simulink model "PMSM_FOC_Average_Inveter"  (R2020b)
settings: Solver=FixedStepAuto  StartTime=0.0  StopTime=10  FixedStep=Fixed_Step_Size  RelTol=1e-3
model workspace (MAT data in the model file):
  wc : Simulink.Parameter (value not decoded)
values from neighbouring files (symbols this model uses):
  Angle = 1.0    [Motor_Control_Data.sldd]
  Cosine_table = 1.0 0.99999529 0.99999058 0.99998587 0.99998116 0.99996704 0.99995291 0.99993885 0.99992472 0.99990118 0.99987763 0.99985409 0.9998306 0.99979764 0.99976468 0.99973178 0.99969882 0.99965644 0.99961412 0.99957174 0.99952942 0.99947762 0.99942589 0.99937415 0.99932235 0.9992612 0.99920005 0.99913889 0.99907768 0.99900717 0.99893659 0.99886602 0.99879545 0.99871546 0.99863547 0.99855554 0.99847555 0.    [Motor_Control_Data.sldd]
  Fixed_Step_Size = 1.0E-5    [Motor_Control_Data.sldd]
  Flux = 0.1125    [Motor_Control_Data.sldd]
  ID_Ki = 48.0    [Motor_Control_Data.sldd]
  ID_Kp = 0.84    [Motor_Control_Data.sldd]
  IQ_Ki = 48.0    [Motor_Control_Data.sldd]
  IQ_Kp = 1.869    [Motor_Control_Data.sldd]
  Ld = 0.00014    [Motor_Control_Data.sldd]
  Lq = 0.0003115    [Motor_Control_Data.sldd]
  MTPA_Te_Min = 0.0    [Motor_Control_Data.sldd]
  Pole_Pairs = 4.0    [Motor_Control_Data.sldd]
  PWM_Frequency = 10000.0    [Motor_Control_Data.sldd]
  Sine_table = 0.0 0.0015339879 0.0030679768 0.0046019657 0.0061359555 0.0076698866 0.0092038177 0.010737749 0.012271681 0.013805497 0.015339312 0.016873131 0.018406944 0.019940587 0.021474229 0.023007872 0.024541514 0.026074925 0.027608337 0.029141748 0.03067516 0.032208283 0.033741407 0.035274528 0.036807653 0.038340431 0.039873205 0.04140598 0.042938754 0.04447113 0.046003502 0.047535874 0.049068246 0.0506001    [Motor_Control_Data.sldd]
  Speed_Ki = 10.809    [Motor_Control_Data.sldd]
  Speed_Kp = 0.08    [Motor_Control_Data.sldd]
  Speed_PI_OutputMax = 700.0    [Motor_Control_Data.sldd]
  Speed_PI_OutputMin = -700.0    [Motor_Control_Data.sldd]
  TorqueMode = 0.0    [Motor_Control_Data.sldd]
undefined symbols (not defined in the file or in its folder): Angle_offset, DiscIntNeverNeededParam, FluxWeak_Enable, FluxWeak_Idref_max, FluxWeak_Idref_min, FluxWeak_Ki, FluxWeak_Kp, inverter, MTPA_id_table, MTPA_iq_table, MTPA_Te_Max, Over_modulation, sigbuilder_block, SVPWM
libraries: simulink x7, pid_lib x1, mcbplantlib x1, autolibpmsminterior x1
(part 2 of 2)

== system PMSM_FOC_Average_Inveter/Motor_Control/Motor_Control_Function/FOC_Control_100us/FOC/Inverse_Park_Transform ==
  D : Inport
  Q : Inport  Port=2
  Sin_Coefficient : Inport  Port=3
  Cos_Coefficient : Inport  Port=4
  Add1 : Sum  Inputs=+-  OutDataTypeStr=Inherit: Same as first input
  Add2 : Sum  OutDataTypeStr=Inherit: Same as first input
  Cos_Coefficient1 : InportShadow  Port=4
  Product{1..4} (4 alike) : Product  RndMeth=Simplest  OutDataTypeStr=Inherit: Same as first input
  Sin_Coefficient1 : InportShadow  Port=3
  Alpha : Outport  VectorParamsAs1DForOutWhenUnconnected=off
  Beta : Outport  Port=2  VectorParamsAs1DForOutWhenUnconnected=off
  wires:
  Add2/1 -> Beta/1
  Add1/1 -> Alpha/1
  Product3/1 -> Add2/1
  Product4/1 -> Add2/2
  Product1/1 -> Add1/1
  Product2/1 -> Add1/2
  Cos_Coefficient1/1 -> Product4/2
  Sin_Coefficient/1 -> Product2/2
  D/1 -> Product3/1, Product1/1
  Q/1 -> Product2/1, Product4/1
  Sin_Coefficient1/1 -> Product3/2
  Cos_Coefficient/1 -> Product1/2

== system PMSM_FOC_Average_Inveter/Motor_Control/Motor_Control_Function/FOC_Control_100us/FOC/Park_Transform ==
  Alpha : Inport
  Beta : Inport  Port=2
  Sin_Coefficient : Inport  Port=3
  Cos_Coefficient : Inport  Port=4
  Add1 : Sum  OutDataTypeStr=Inherit: Same as first input
  Add2 : Sum  Inputs=-+  OutDataTypeStr=Inherit: Same as first input
  Alpha1 : InportShadow
  Beta1 : InportShadow  Port=2
  Cos_Coefficient1 : InportShadow  Port=4
  Produc3t : Product  RndMeth=Simplest  OutDataTypeStr=Inherit: Same as first input
  Product1 : Product  RndMeth=Simplest  OutDataTypeStr=Inherit: Same as first input
  Product2 : Product  RndMeth=Simplest  OutDataTypeStr=Inherit: Same as first input
  Product4 : Product  RndMeth=Simplest  OutDataTypeStr=Inherit: Same as first input
  Sin_Coefficient1 : InportShadow  Port=3
  D : Outport  VectorParamsAs1DForOutWhenUnconnected=off
  Q : Outport  Port=2  VectorParamsAs1DForOutWhenUnconnected=off
  wires:
  Produc3t/1 -> Add2/1
  Product4/1 -> Add2/2
  Product1/1 -> Add1/1
  Product2/1 -> Add1/2
  Alpha1/1 -> Produc3t/1
  Sin_Coefficient1/1 -> Produc3t/2
  Cos_Coefficient1/1 -> Product4/2
  Beta1/1 -> Product4/1
  Alpha/1 -> Product1/1
  Cos_Coefficient/1 -> Product1/2
  Beta/1 -> Product2/1
  Sin_Coefficient/1 -> Product2/2
  Add1/1 -> D/1
  Add2/1 -> Q/1

== system PMSM_FOC_Average_Inveter/Motor_Control/Motor_Control_Function/FOC_Control_100us/FOC/Q_Current_PI ==
  Reset : Inport
  Bus_voltage : Inport  Port=2
  Current_Command : Inport  Port=3
  Current_Measured : Inport  Port=4
  Add2 : Sum  Inputs=|+-
  IQ_Control : Subsystem
  Vq_voltage : Outport  VectorParamsAs1DForOutWhenUnconnected=off
  wires:
  Current_Command/1 -> Add2/1
  Current_Measured/1 -> Add2/2
  Add2/1 -> IQ_Control/3(Err)  "currentControlError"
  IQ_Control/1(PI_Out) -> Vq_voltage/1
  Reset/1 -> IQ_Control/1(Reset)
  Bus_voltage/1 -> IQ_Control/2(Bus_voltage)

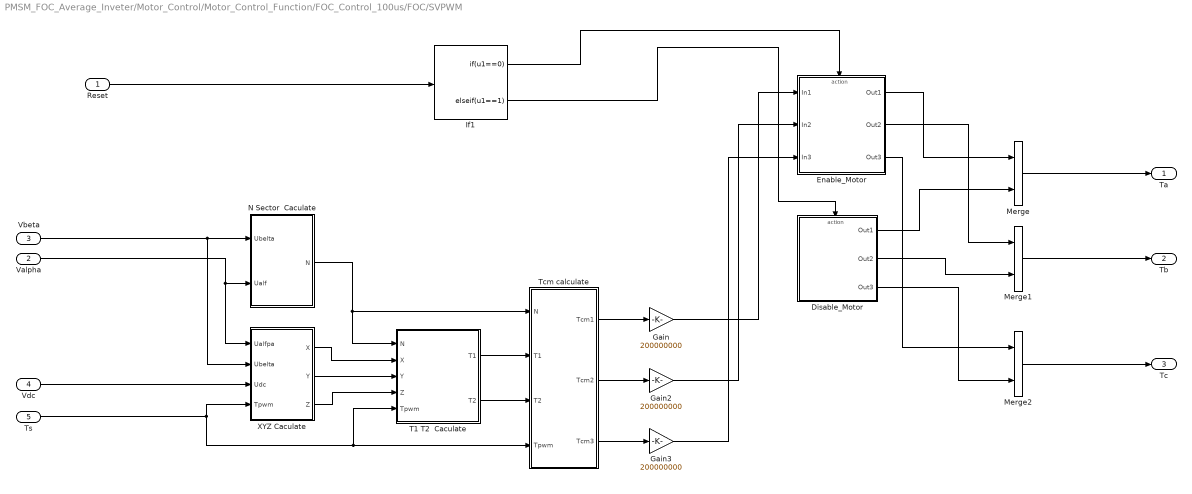
== system PMSM_FOC_Average_Inveter/Motor_Control/Motor_Control_Function/FOC_Control_100us/FOC/SVPWM ==
  Reset : Inport
  Valpha : Inport  Port=2
  Vbeta : Inport  Port=3
  Vdc : Inport  Port=4
  Ts : Inport  Port=5
  Disable_Motor : Subsystem  TreatAsAtomicUnit=on
  Enable_Motor : Subsystem  TreatAsAtomicUnit=on
  Gain : Gain  Gain=200000000
  Gain2 : Gain  Gain=200000000
  Gain3 : Gain  Gain=200000000
  If1 : If  IfExpression=u1==0  ElseIfExpressions=u1==1  ShowElse=off
  Merge : Merge
  Merge1 : Merge
  Merge2 : Merge
  N Sector  Caculate : Subsystem  TreatAsAtomicUnit=on
  T1 T2  Caculate : Subsystem  TreatAsAtomicUnit=on
  Tcm calculate : Subsystem  TreatAsAtomicUnit=on
  XYZ Caculate : Subsystem  TreatAsAtomicUnit=on
  Ta : Outport
  Tb : Outport  Port=2
  Tc : Outport  Port=3
  wires:
  Tcm calculate/2(Tcm2) -> Gain2/1
  Tcm calculate/3(Tcm3) -> Gain3/1
  Tcm calculate/1(Tcm1) -> Gain/1
  T1 T2  Caculate/2(T2) -> Tcm calculate/3(T2)
  XYZ Caculate/1(X) -> T1 T2  Caculate/2(X)
  N Sector  Caculate/1(N) -> T1 T2  Caculate/1(N), Tcm calculate/1(N)
  Vdc/1 -> XYZ Caculate/3(Udc)
  T1 T2  Caculate/1(T1) -> Tcm calculate/2(T1)
  XYZ Caculate/3(Z) -> T1 T2  Caculate/4(Z)
  XYZ Caculate/2(Y) -> T1 T2  Caculate/3(Y)
  Valpha/1 -> N Sector  Caculate/2(Ualf), XYZ Caculate/1(Ualfpa)
  Vbeta/1 -> N Sector  Caculate/1(Ubelta), XYZ Caculate/2(Ubelta)
  Ts/1 -> T1 T2  Caculate/5(Tpwm), Tcm calculate/4(Tpwm), XYZ Caculate/4(Tpwm)
  Gain/1 -> Enable_Motor/1(In1)
  Gain2/1 -> Enable_Motor/2(In2)
  Reset/1 -> If1/1
  If1/1 -> Enable_Motor/Action
  If1/2 -> Disable_Motor/Action
  Gain3/1 -> Enable_Motor/3(In3)
  Enable_Motor/1(Out1) -> Merge/1
  Disable_Motor/1(Out1) -> Merge/2
  Enable_Motor/2(Out2) -> Merge1/1
  Disable_Motor/2(Out2) -> Merge1/2
  Enable_Motor/3(Out3) -> Merge2/1
  Disable_Motor/3(Out3) -> Merge2/2
  Merge/1 -> Ta/1
  Merge1/1 -> Tb/1
  Merge2/1 -> Tc/1

== system PMSM_FOC_Average_Inveter/Motor_Control/Motor_Control_Function/FOC_Control_100us/FOC/Sine_Cosine ==
  note: Sine Cosine Coefficients
  P : Inport
  Cosine : Lookup_n-D  NumberOfTableDimensions=1  LookupTableObject=''  BreakpointsForDimension1=[0:2*pi/4095:2*pi]  BreakpointsForDimension1FirstPoint=10  BreakpointsForDimension2FirstPoint=10  BreakpointsForDimension1Spacing=12  BreakpointsForDimension2Spacing=12  IndexSearchMethod=Evenly spaced points  Table=Cosine_table  InterpMethod=Flat  DiagnosticForOutOfRangeInput=Error  InternalRulePriority=Speed  RndMeth=Simplest  InputSameDT=on
  Saturation : Saturate  UpperLimit=2*pi-0.0001  LowerLimit=0+0.0001
  Scope : Scope  NumInputPorts=2
  Sine : Lookup_n-D  NumberOfTableDimensions=1  LookupTableObject=''  BreakpointsForDimension1=[0:2*pi/4095:2*pi]  BreakpointsForDimension1FirstPoint=10  BreakpointsForDimension2FirstPoint=10  BreakpointsForDimension1Spacing=12  BreakpointsForDimension2Spacing=12  IndexSearchMethod=Evenly spaced points  Table=Sine_table  InterpMethod=Flat  DiagnosticForOutOfRangeInput=Error  InternalRulePriority=Speed  RndMeth=Simplest  InputSameDT=on
  Sin : Outport  VectorParamsAs1DForOutWhenUnconnected=off
  Cos : Outport  Port=2  VectorParamsAs1DForOutWhenUnconnected=off
  wires:
  P/1 -> Saturation/1  "position"
  Sine/1 -> Scope/1, Sin/1
  Cosine/1 -> Scope/2, Cos/1
  Saturation/1 -> Cosine/1, Sine/1

== system PMSM_FOC_Average_Inveter/Motor_Control/Motor_Control_Function/SYM_State_10ms/Bus_voltage/Normal_Voltage ==
  Action Port : ActionPort
  Constant : Constant  Value=2  OutDataTypeStr=uint8
  Normal_Voltage : Outport  VectorParamsAs1DForOutWhenUnconnected=off
  wires:
  Constant/1 -> Normal_Voltage/1

== system PMSM_FOC_Average_Inveter/Motor_Control/Motor_Control_Function/SYM_State_10ms/Bus_voltage/Over_Voltage ==
  Action Port : ActionPort
  Constant : Constant  Value=0  OutDataTypeStr=uint8
  Over_voltage : Outport  VectorParamsAs1DForOutWhenUnconnected=off
  wires:
  Constant/1 -> Over_voltage/1

== system PMSM_FOC_Average_Inveter/Motor_Control/Motor_Control_Function/SYM_State_10ms/Bus_voltage/Under_Voltage ==
  Action Port : ActionPort
  Constant : Constant  OutDataTypeStr=uint8
  Under_voltage : Outport  VectorParamsAs1DForOutWhenUnconnected=off
  wires:
  Constant/1 -> Under_voltage/1

== system PMSM_FOC_Average_Inveter/Motor_Control/Motor_Control_Function/Angle_Speed_100us/Resolver_Observer/Angle_calibration/If Action Subsystem1 ==
  In1 : Inport
  Action Port : ActionPort
  Out1 : Outport
  wires:
  In1/1 -> Out1/1

== system PMSM_FOC_Average_Inveter/Motor_Control/Motor_Control_Function/Angle_Speed_100us/Resolver_Observer/Angle_calibration/If Action Subsystem2 ==
  In1 : Inport
  Action Port : ActionPort
  2pi : Constant  Value=2*pi  OutDataTypeStr=single
  Subtract1 : Sum  Inputs=+-
  Out1 : Outport
  wires:
  In1/1 -> Subtract1/1
  Subtract1/1 -> Out1/1
  2pi/1 -> Subtract1/2

== system PMSM_FOC_Average_Inveter/Motor_Control/Motor_Control_Function/Angle_Speed_100us/Resolver_Observer/Resolver_Angle_cacl/Sine_Cosine ==
  note: Sine Cosine Coefficients
  P : Inport
  Cosine : Lookup_n-D  NumberOfTableDimensions=1  LookupTableObject=''  BreakpointsForDimension1=[0:2*pi/4095:2*pi]  BreakpointsForDimension1FirstPoint=10  BreakpointsForDimension2FirstPoint=10  BreakpointsForDimension1Spacing=12  BreakpointsForDimension2Spacing=12  IndexSearchMethod=Evenly spaced points  Table=Cosine_table  InterpMethod=Flat  DiagnosticForOutOfRangeInput=Error  InternalRulePriority=Speed  RndMeth=Simplest  InputSameDT=on
  Saturation : Saturate  UpperLimit=2*pi-0.0001  LowerLimit=0+0.0001
  Scope : Scope  NumInputPorts=2
  Sine : Lookup_n-D  NumberOfTableDimensions=1  LookupTableObject=''  BreakpointsForDimension1=[0:2*pi/4095:2*pi]  BreakpointsForDimension1FirstPoint=10  BreakpointsForDimension2FirstPoint=10  BreakpointsForDimension1Spacing=12  BreakpointsForDimension2Spacing=12  IndexSearchMethod=Evenly spaced points  Table=Sine_table  InterpMethod=Flat  DiagnosticForOutOfRangeInput=Error  InternalRulePriority=Speed  RndMeth=Simplest  InputSameDT=on
  Sin : Outport  VectorParamsAs1DForOutWhenUnconnected=off
  Cos : Outport  Port=2  VectorParamsAs1DForOutWhenUnconnected=off
  wires:
  P/1 -> Saturation/1  "position"
  Sine/1 -> Scope/1, Sin/1
  Cosine/1 -> Scope/2, Cos/1
  Saturation/1 -> Cosine/1, Sine/1

== system PMSM_FOC_Average_Inveter/Motor_Control/Motor_Control_Function/Control_Command_2ms/Control_Command_2ms/Speed_PI/Speed_PI ==
  PI_input : Inport
  Reset : Inport  Port=2
  Speed_Control : Subsystem
  PI_out : Outport  VectorParamsAs1DForOutWhenUnconnected=off
  wires:
  PI_input/1 -> Speed_Control/1(Err)
  Speed_Control/1(PI_Out) -> PI_out/1
  Reset/1 -> Speed_Control/2(Reset)

== system PMSM_FOC_Average_Inveter/Motor_Control/Motor_Control_Function/FOC_Control_100us/FOC/Clarke_Transform/Clark1 ==
  Iabc : Inport
  Add : Sum  Inputs=+--
  Add1 : Sum  Inputs=+-
  Demux : Demux  Outputs=3
  Gain : Gain  Gain=0.5
  Gain1 : Gain  Gain=0.5
  Gain2 : Gain  Gain=sqrt(2/3)
  Gain3 : Gain  Gain=sqrt(3)/2
  Gain4 : Gain  Gain=sqrt(3)/2
  Gain5 : Gain  Gain=sqrt(2/3)
  Ialpha : Outport  VectorParamsAs1DForOutWhenUnconnected=off
  Ibeta : Outport  Port=2  VectorParamsAs1DForOutWhenUnconnected=off
  wires:
  Iabc/1 -> Demux/1
  Demux/1 -> Add/1
  Gain/1 -> Add/2
  Demux/2 -> Gain3/1, Gain/1
  Gain1/1 -> Add/3
  Demux/3 -> Gain4/1, Gain1/1
  Add/1 -> Gain2/1
  Gain2/1 -> Ialpha/1
  Gain3/1 -> Add1/1
  Gain4/1 -> Add1/2
  Add1/1 -> Gain5/1
  Gain5/1 -> Ibeta/1

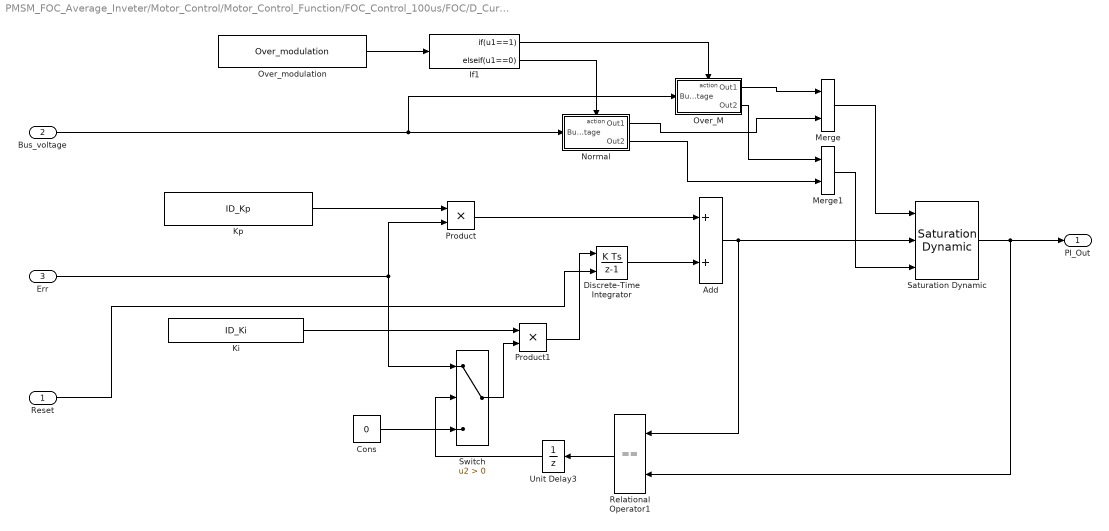
== system PMSM_FOC_Average_Inveter/Motor_Control/Motor_Control_Function/FOC_Control_100us/FOC/D_Current_PI/ID_Control ==
  Reset : Inport
  Bus_voltage : Inport  Port=2
  Err : Inport  Port=3
  Add : Sum
  Cons : Constant  Value=0  OutDataTypeStr=single
  Discrete-Time Integrator : DiscreteIntegrator  ExternalReset=level  SampleTime=-1  ICPrevOutput=DiscIntNeverNeededParam  ICPrevScaledInput=DiscIntNeverNeededParam
  If1 : If  IfExpression=u1==1  ElseIfExpressions=u1==0  ShowElse=off
  Ki : Constant  Value=ID_Ki  OutDataTypeStr=single
  Kp : Constant  Value=ID_Kp  OutDataTypeStr=single
  Merge : Merge
  Merge1 : Merge
  Normal : Subsystem  TreatAsAtomicUnit=on
  Over_M : Subsystem  TreatAsAtomicUnit=on
  Over_modulation : Constant  Value=Over_modulation  OutDataTypeStr=boolean
  Product : Product
  Product1 : Product
  Relational Operator1 : RelationalOperator  Operator===  OutDataTypeStr=boolean  RndMeth=Simplest
  Saturation Dynamic : simulink/Discontinuities/Saturation Dynamic  OutMin=[]  OutMax=[]  OutDataTypeStr=Inherit: Same as second input  OutDataType=fixdt(1, 16)  OutScaling=2^-10  DoSatur=off
  Switch : Switch  Criteria=u2 > Threshold
  Unit Delay3 : UnitDelay  SampleTime=-1  HasFrameUpgradeWarning=on
  PI_Out : Outport
  wires:
  Kp/1 -> Product/1
  Err/1 -> Product/2, Switch/1
  Switch/1 -> Product1/2
  Product1/1 -> Discrete-Time Integrator/1
  Product/1 -> Add/1
  Add/1 -> Saturation Dynamic/2, Relational Operator1/1
  Saturation Dynamic/1 -> Relational Operator1/2, PI_Out/1
  Cons/1 -> Switch/3
  Discrete-Time Integrator/1 -> Add/2
  Relational Operator1/1 -> Unit Delay3/1
  Ki/1 -> Product1/1
  Unit Delay3/1 -> Switch/2
  Reset/1 -> Discrete-Time Integrator/2
  Over_modulation/1 -> If1/1
  If1/2 -> Normal/Action
  If1/1 -> Over_M/Action
  Bus_voltage/1 -> Over_M/1(Bus_voltage), Normal/1(Bus_voltage)
  Over_M/1(Out1) -> Merge/1
  Normal/1(Out1) -> Merge/2
  Over_M/2(Out2) -> Merge1/1
  Normal/2(Out2) -> Merge1/2
  Merge/1 -> Saturation Dynamic/1
  Merge1/1 -> Saturation Dynamic/3

== system PMSM_FOC_Average_Inveter/Motor_Control/Motor_Control_Function/FOC_Control_100us/FOC/Flux_weakening /Subsystem ==
  Reset : Inport
  Vd : Inport  Port=2
  Vq : Inport  Port=3
  Id : Inport  Port=4
  Iq : Inport  Port=5
  Bus_voltage : Inport  Port=6
  Action Port : ActionPort
  Flux_weak : Subsystem  TreatAsAtomicUnit=on  mask{kp=FluxWeak_Kp, ki=FluxWeak_Ki, Id_max=FluxWeak_Idref_max, Id_min=FluxWeak_Idref_min}
      settings: RTWSystemCode=Nonreusable function  RTWFcnNameOpts=Use subsystem name
  Id_ref : Outport
  Iq_ref : Outport  Port=2
  wires:
  Vd/1 -> Flux_weak/2(Vd)
  Vq/1 -> Flux_weak/3(Vq)
  Id/1 -> Flux_weak/4(id_input)
  Iq/1 -> Flux_weak/5(Iq_input)
  Flux_weak/1(Id_ref) -> Id_ref/1
  Flux_weak/2(iq_ref) -> Iq_ref/1
  Reset/1 -> Flux_weak/1(Reset)
  Bus_voltage/1 -> Flux_weak/6(Bus_voltage)

== system PMSM_FOC_Average_Inveter/Motor_Control/Motor_Control_Function/FOC_Control_100us/FOC/Flux_weakening /Subsystem1 ==
  Id : Inport
  Iq : Inport  Port=2
  Action Port : ActionPort
  Id_ref : Outport
  Iq_ref : Outport  Port=2
  wires:
  Id/1 -> Id_ref/1
  Iq/1 -> Iq_ref/1

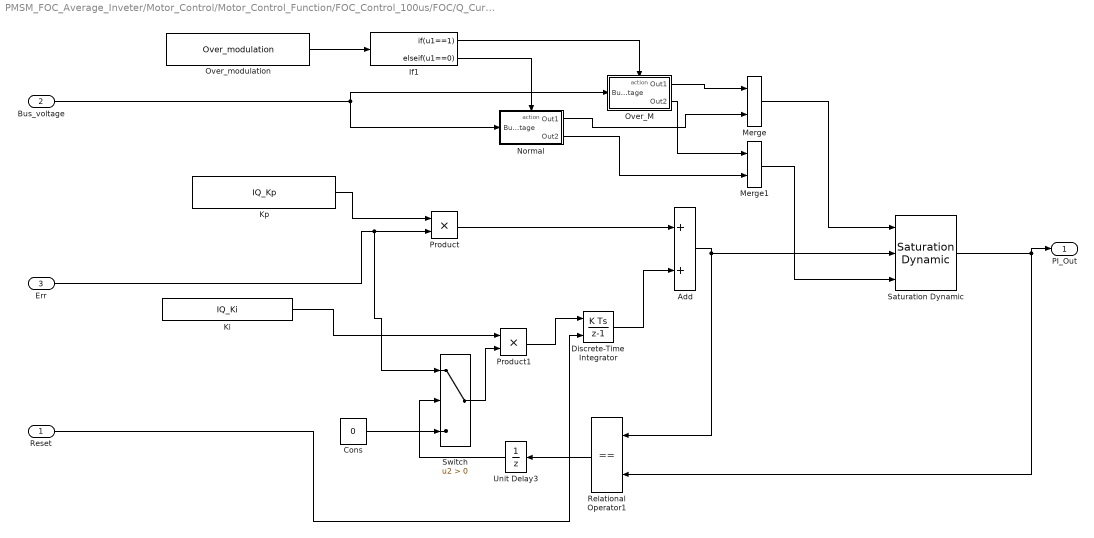
== system PMSM_FOC_Average_Inveter/Motor_Control/Motor_Control_Function/FOC_Control_100us/FOC/Q_Current_PI/IQ_Control ==
  Reset : Inport
  Bus_voltage : Inport  Port=2
  Err : Inport  Port=3
  Add : Sum
  Cons : Constant  Value=0  OutDataTypeStr=single
  Discrete-Time Integrator : DiscreteIntegrator  ExternalReset=level  SampleTime=-1  ICPrevOutput=DiscIntNeverNeededParam  ICPrevScaledInput=DiscIntNeverNeededParam
  If1 : If  IfExpression=u1==1  ElseIfExpressions=u1==0  ShowElse=off
  Ki : Constant  Value=IQ_Ki  OutDataTypeStr=single
  Kp : Constant  Value=IQ_Kp  OutDataTypeStr=single
  Merge : Merge
  Merge1 : Merge
  Normal : Subsystem  TreatAsAtomicUnit=on
  Over_M : Subsystem  TreatAsAtomicUnit=on
  Over_modulation : Constant  Value=Over_modulation  OutDataTypeStr=boolean
  Product : Product
  Product1 : Product
  Relational Operator1 : RelationalOperator  Operator===  OutDataTypeStr=boolean  RndMeth=Simplest
  Saturation Dynamic : simulink/Discontinuities/Saturation Dynamic  OutMin=[]  OutMax=[]  OutDataTypeStr=Inherit: Same as second input  OutDataType=fixdt(1, 16)  OutScaling=2^-10  DoSatur=off
  Switch : Switch  Criteria=u2 > Threshold
  Unit Delay3 : UnitDelay  SampleTime=-1  HasFrameUpgradeWarning=on
  PI_Out : Outport
  wires:
  Kp/1 -> Product/1
  Err/1 -> Switch/1, Product/2
  Switch/1 -> Product1/2
  Product1/1 -> Discrete-Time Integrator/1
  Product/1 -> Add/1
  Add/1 -> Saturation Dynamic/2, Relational Operator1/1
  Saturation Dynamic/1 -> PI_Out/1, Relational Operator1/2
  Cons/1 -> Switch/3
  Discrete-Time Integrator/1 -> Add/2
  Relational Operator1/1 -> Unit Delay3/1
  Ki/1 -> Product1/1
  Unit Delay3/1 -> Switch/2
  Reset/1 -> Discrete-Time Integrator/2
  Normal/1(Out1) -> Merge/2
  Over_M/1(Out1) -> Merge/1
  Over_modulation/1 -> If1/1
  Normal/2(Out2) -> Merge1/2
  If1/2 -> Normal/Action
  Bus_voltage/1 -> Normal/1(Bus_voltage), Over_M/1(Bus_voltage)
  If1/1 -> Over_M/Action
  Over_M/2(Out2) -> Merge1/1
  Merge/1 -> Saturation Dynamic/1
  Merge1/1 -> Saturation Dynamic/3

== system PMSM_FOC_Average_Inveter/Motor_Control/Motor_Control_Function/FOC_Control_100us/FOC/SVPWM/Disable_Motor ==
  Action Port : ActionPort
  Constant : Constant  Value=0  OutDataTypeStr=single
  Constant1 : Constant  Value=0  OutDataTypeStr=single
  Constant2 : Constant  Value=0  OutDataTypeStr=single
  Out1 : Outport
  Out2 : Outport  Port=2
  Out3 : Outport  Port=3
  wires:
  Constant/1 -> Out1/1
  Constant1/1 -> Out2/1
  Constant2/1 -> Out3/1

== system PMSM_FOC_Average_Inveter/Motor_Control/Motor_Control_Function/FOC_Control_100us/FOC/SVPWM/Enable_Motor ==
  In1 : Inport
  In2 : Inport  Port=2
  In3 : Inport  Port=3
  Action Port : ActionPort
  Out1 : Outport
  Out2 : Outport  Port=2
  Out3 : Outport  Port=3
  wires:
  In1/1 -> Out1/1
  In2/1 -> Out2/1
  In3/1 -> Out3/1

== system PMSM_FOC_Average_Inveter/Motor_Control/Motor_Control_Function/FOC_Control_100us/FOC/SVPWM/N Sector  Caculate ==
  Ubelta : Inport
  Ualf : Inport  Port=2
  Add : Sum  Inputs=+++
  Add1 : Sum  Inputs=-+
  Add2 : Sum  Inputs=--
  Constant : Constant  OutDataTypeStr=single
  Constant1 : Constant  Value=0  OutDataTypeStr=single
  Gain : Gain  Gain=sqrt(3)
  Gain1 : Gain  Gain=2
  Gain2 : Gain  Gain=4
  Saturation : Saturate  UpperLimit=6  LowerLimit=1
  Switch : Switch
  Switch1 : Switch
  Switch2 : Switch
  N : Outport
  wires:
  Saturation/1 -> N/1
  Add/1 -> Saturation/1
  Gain2/1 -> Add/3
  Switch2/1 -> Gain2/1
  Add2/1 -> Switch2/2
  Gain1/1 -> Add/2
  Switch1/1 -> Gain1/1
  Add1/1 -> Switch1/2
  Gain/1 -> Add2/2, Add1/2
  Ualf/1 -> Gain/1
  Switch/1 -> Add/1
  Constant1/1 -> Switch/3, Switch1/3, Switch2/3
  Constant/1 -> Switch/1, Switch1/1, Switch2/1
  Ubelta/1 -> Add2/1, Add1/1, Switch/2

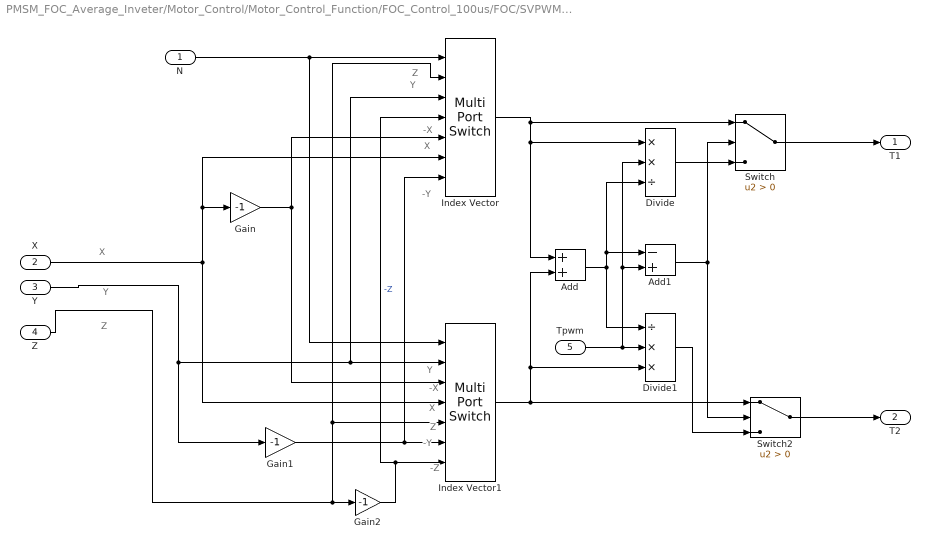
== system PMSM_FOC_Average_Inveter/Motor_Control/Motor_Control_Function/FOC_Control_100us/FOC/SVPWM/T1 T2  Caculate ==
  note: Z
  note: Y
  note: -X
  note: X
  note: -Y
  note: Y
  note: -X
  note: X
  note: Z
  note: -Y
  note: -Z
  note: X
  note: Y
  note: Z
  N : Inport
  X : Inport  Port=2
  Y : Inport  Port=3
  Z : Inport  Port=4
  Tpwm : Inport  Port=5
  Add : Sum
  Add1 : Sum  Inputs=-+
  Divide : Product  Inputs=**/
  Divide1 : Product  Inputs=/**
  Gain : Gain  Gain=-1
  Gain1 : Gain  Gain=-1
  Gain2 : Gain  Gain=-1
  Index Vector : MultiPortSwitch  Inputs=6
  Index Vector1 : MultiPortSwitch  Inputs=6
  Switch : Switch  Criteria=u2 > Threshold
  Switch2 : Switch  Criteria=u2 > Threshold
  T1 : Outport
  T2 : Outport  Port=2
  wires:
  Switch2/1 -> T2/1
  Divide1/1 -> Switch2/3
  Switch/1 -> T1/1
  Add1/1 -> Switch/2, Switch2/2
  Add/1 -> Divide1/1, Divide/3, Add1/1
  Tpwm/1 -> Divide1/2, Divide/2, Add1/2
  Divide/1 -> Switch/3
  Index Vector1/1 -> Switch2/1, Add/2, Divide1/3
  Index Vector/1 -> Switch/1, Divide/1, Add/1
  Gain1/1 -> Index Vector/7, Index Vector1/6
  Gain2/1 -> Index Vector/4, Index Vector1/7  "-Z"
  Gain/1 -> Index Vector/5, Index Vector1/3
  Y/1 -> Gain1/1, Index Vector/3, Index Vector1/2
  X/1 -> Index Vector1/4, Index Vector/6, Gain/1
  Z/1 -> Index Vector/2, Index Vector1/5, Gain2/1
  N/1 -> Index Vector1/1, Index Vector/1

== system PMSM_FOC_Average_Inveter/Motor_Control/Motor_Control_Function/FOC_Control_100us/FOC/SVPWM/Tcm calculate ==
  note: Tc
  note: Tb
  note: Ta
  N : Inport
  T1 : Inport  Port=2
  T2 : Inport  Port=3
  Tpwm : Inport  Port=4
  Add : Sum  Inputs=--+
  Add1 : Sum
  Add2 : Sum
  Gain : Gain  Gain=0.5
  Gain1 : Gain  Gain=0.5
  Gain2 : Gain  Gain=1/4
  Index Vector : MultiPortSwitch  Inputs=6
  Index Vector1 : MultiPortSwitch  Inputs=6
  Index Vector2 : MultiPortSwitch  Inputs=6
  Scope2 : Scope  NumInputPorts=3
  Tcm1 : Outport
  Tcm2 : Outport  Port=2
  Tcm3 : Outport  Port=3
  wires:
  Index Vector2/1 -> Scope2/3, Tcm3/1
  N/1 -> Index Vector/1, Index Vector1/1, Index Vector2/1
  Add2/1 -> Index Vector/5, Index Vector/6, Index Vector1/3, Index Vector1/7, Index Vector2/2, Index Vector2/4
  Gain1/1 -> Add2/1
  Add1/1 -> Add2/2, Index Vector/2, Index Vector/7, Index Vector1/4, Index Vector1/5, Index Vector2/3, Index Vector2/6
  Gain2/1 -> Index Vector2/5, Index Vector2/7, Add1/2, Index Vector/3, Index Vector/4, Index Vector1/2, Index Vector1/6
  Gain/1 -> Add1/1
  Add/1 -> Gain2/1
  Tpwm/1 -> Add/3
  T2/1 -> Add/2, Gain1/1
  T1/1 -> Add/1, Gain/1
  Index Vector/1 -> Scope2/1, Tcm1/1
  Index Vector1/1 -> Scope2/2, Tcm2/1

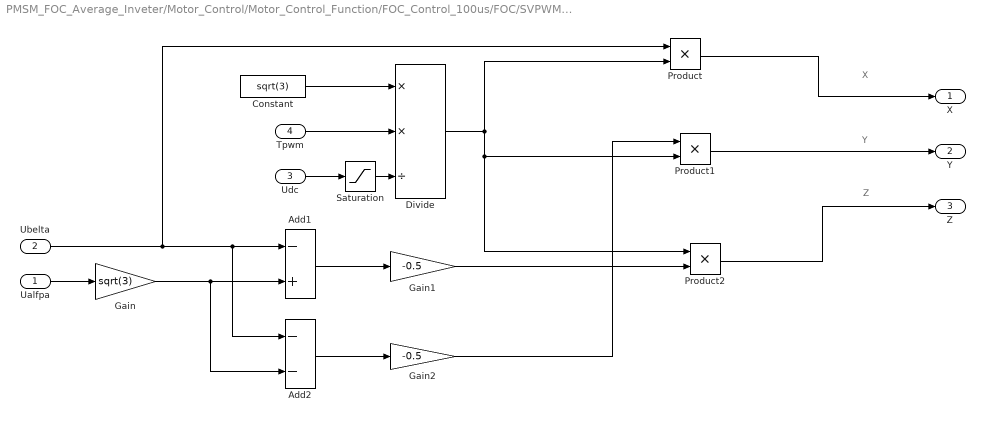
== system PMSM_FOC_Average_Inveter/Motor_Control/Motor_Control_Function/FOC_Control_100us/FOC/SVPWM/XYZ Caculate ==
  note: X
  note: Y
  note: Z
  Ualfpa : Inport
  Ubelta : Inport  Port=2
  Udc : Inport  Port=3
  Tpwm : Inport  Port=4
  Add1 : Sum  Inputs=-+
  Add2 : Sum  Inputs=--
  Constant : Constant  Value=sqrt(3)  OutDataTypeStr=single
  Divide : Product  Inputs=**/
  Gain : Gain  Gain=sqrt(3)
  Gain1 : Gain  Gain=-0.5
  Gain2 : Gain  Gain=-0.5
  Product : Product
  Product1 : Product
  Product2 : Product
  Saturation : Saturate  UpperLimit=1200  LowerLimit=0.0001
  X : Outport
  Y : Outport  Port=2
  Z : Outport  Port=3
  wires:
  Gain2/1 -> Product1/1
  Add2/1 -> Gain2/1
  Add1/1 -> Gain1/1
  Gain/1 -> Add2/2, Add1/2
  Ualfpa/1 -> Gain/1
  Ubelta/1 -> Add2/1, Add1/1, Product/1
  Gain1/1 -> Product2/2
  Product2/1 -> Z/1
  Divide/1 -> Product1/2, Product2/1, Product/2
  Product1/1 -> Y/1
  Product/1 -> X/1
  Udc/1 -> Saturation/1
  Tpwm/1 -> Divide/2
  Constant/1 -> Divide/1
  Saturation/1 -> Divide/3

== system PMSM_FOC_Average_Inveter/Motor_Control/Motor_Control_Function/Control_Command_2ms/Control_Command_2ms/Speed_PI/Speed_PI/Speed_Control ==
  Err : Inport
  Reset : Inport  Port=2
  Add : Sum
  Cons : Constant  Value=0  OutDataTypeStr=single
  Discrete-Time Integrator : DiscreteIntegrator  ExternalReset=level  SampleTime=-1  ICPrevOutput=DiscIntNeverNeededParam  ICPrevScaledInput=DiscIntNeverNeededParam
  Ki : Constant  Value=Speed_Ki  OutDataTypeStr=single
  Kp : Constant  Value=Speed_Kp  OutDataTypeStr=single
  Product : Product
  Product1 : Product
  Relational Operator1 : RelationalOperator  Operator===  OutDataTypeStr=boolean  RndMeth=Simplest
  Saturation : Saturate  UpperLimit=Speed_PI_OutputMax  LowerLimit=Speed_PI_OutputMin
  Scope : Scope
  Switch : Switch  Criteria=u2 > Threshold
  Unit Delay3 : UnitDelay  SampleTime=-1  HasFrameUpgradeWarning=on
  PI_Out : Outport
  wires:
  Kp/1 -> Product/1
  Err/1 -> Switch/1, Product/2
  Switch/1 -> Product1/2
  Product1/1 -> Discrete-Time Integrator/1
  Product/1 -> Add/1
  Add/1 -> Relational Operator1/1, Saturation/1
  Saturation/1 -> Relational Operator1/2, PI_Out/1
  Discrete-Time Integrator/1 -> Add/2, Scope/1
  Relational Operator1/1 -> Unit Delay3/1
  Ki/1 -> Product1/1
  Unit Delay3/1 -> Switch/2
  Cons/1 -> Switch/3
  Reset/1 -> Discrete-Time Integrator/2

== system PMSM_FOC_Average_Inveter/Motor_Control/Motor_Control_Function/FOC_Control_100us/FOC/D_Current_PI/ID_Control/Normal ==
  Bus_voltage : Inport
  Action Port : ActionPort
  Gain : Gain  Gain=1/sqrt(3)
  Gain1 : Gain  Gain=-1/sqrt(3)
  Out1 : Outport
  Out2 : Outport  Port=2
  wires:
  Bus_voltage/1 -> Gain1/1, Gain/1
  Gain/1 -> Out1/1
  Gain1/1 -> Out2/1

== system PMSM_FOC_Average_Inveter/Motor_Control/Motor_Control_Function/FOC_Control_100us/FOC/D_Current_PI/ID_Control/Over_M ==
  Bus_voltage : Inport
  Action Port : ActionPort
  Gain : Gain  Gain=2/3
  Gain1 : Gain  Gain=-2/3
  Out1 : Outport
  Out2 : Outport  Port=2
  wires:
  Bus_voltage/1 -> Gain1/1, Gain/1
  Gain/1 -> Out1/1
  Gain1/1 -> Out2/1

== system PMSM_FOC_Average_Inveter/Motor_Control/Motor_Control_Function/FOC_Control_100us/FOC/Flux_weakening /Subsystem/Flux_weak ==
  note: sqrt(Ud*Ud+Uq*Uq)<=Udc/sqrt(3)
  Reset : Inport
  Vd : Inport  Port=2
  Vq : Inport  Port=3
  id_input : Inport  Port=4
  Iq_input : Inport  Port=5
  Bus_voltage : Inport  Port=6
  Add1 : Sum  OutDataTypeStr=Inherit: Same as first input
  Fcn : Fcn  Expr=sqrt(u(1)^2+u(2)^2)
  Gain : Gain  Gain=1/sqrt(3)
  ID_Control : Subsystem
  Mux : Mux  Inputs=2
  Sum1 : Sum  Inputs=|-+
  Id_ref : Outport
  iq_ref : Outport  Port=2
  wires:
  Gain/1 -> Sum1/2
  Sum1/1 -> ID_Control/1(Err)
  Mux/1 -> Fcn/1
  Fcn/1 -> Sum1/1
  Vq/1 -> Mux/2
  Iq_input/1 -> iq_ref/1
  id_input/1 -> Add1/1
  Vd/1 -> Mux/1
  Add1/1 -> Id_ref/1
  ID_Control/1(PI_Out) -> Add1/2
  Reset/1 -> ID_Control/2(Reset)
  Bus_voltage/1 -> Gain/1

== system PMSM_FOC_Average_Inveter/Motor_Control/Motor_Control_Function/FOC_Control_100us/FOC/Q_Current_PI/IQ_Control/Normal ==
  Bus_voltage : Inport
  Action Port : ActionPort
  Gain : Gain  Gain=1/sqrt(3)
  Gain1 : Gain  Gain=-1/sqrt(3)
  Out1 : Outport
  Out2 : Outport  Port=2
  wires:
  Bus_voltage/1 -> Gain1/1, Gain/1
  Gain/1 -> Out1/1
  Gain1/1 -> Out2/1

== system PMSM_FOC_Average_Inveter/Motor_Control/Motor_Control_Function/FOC_Control_100us/FOC/Q_Current_PI/IQ_Control/Over_M ==
  Bus_voltage : Inport
  Action Port : ActionPort
  Gain : Gain  Gain=2/3
  Gain1 : Gain  Gain=-2/3
  Out1 : Outport
  Out2 : Outport  Port=2
  wires:
  Bus_voltage/1 -> Gain1/1, Gain/1
  Gain/1 -> Out1/1
  Gain1/1 -> Out2/1

== system PMSM_FOC_Average_Inveter/Motor_Control/Motor_Control_Function/FOC_Control_100us/FOC/Flux_weakening /Subsystem/Flux_weak/ID_Control ==
  Err : Inport
  Reset : Inport  Port=2
  Add : Sum
  Cons : Constant  Value=0  OutDataTypeStr=single
  Discrete-Time Integrator : DiscreteIntegrator  ExternalReset=level  SampleTime=-1  ICPrevOutput=DiscIntNeverNeededParam  ICPrevScaledInput=DiscIntNeverNeededParam
  Ki : Constant  Value=ki  OutDataTypeStr=single
  Kp : Constant  Value=kp  OutDataTypeStr=single
  Product : Product
  Product1 : Product
  Relational Operator1 : RelationalOperator  Operator===  OutDataTypeStr=boolean  RndMeth=Simplest
  Saturation : Saturate  UpperLimit=Id_max  LowerLimit=Id_min
  Switch : Switch  Criteria=u2 > Threshold
  Unit Delay3 : UnitDelay  SampleTime=-1  HasFrameUpgradeWarning=on
  PI_Out : Outport
  wires:
  Kp/1 -> Product/1
  Err/1 -> Switch/1, Product/2
  Switch/1 -> Product1/2
  Product1/1 -> Discrete-Time Integrator/1
  Product/1 -> Add/1
  Add/1 -> Relational Operator1/1, Saturation/1
  Saturation/1 -> Relational Operator1/2, PI_Out/1
  Cons/1 -> Switch/3
  Discrete-Time Integrator/1 -> Add/2
  Relational Operator1/1 -> Unit Delay3/1
  Ki/1 -> Product1/1
  Unit Delay3/1 -> Switch/2
  Reset/1 -> Discrete-Time Integrator/2

== stateflow chart PMSM_FOC_Average_Inveter/Motor_Control/Motor_Control_Function/SYM_State_10ms/Traction_SYM ==
  state Drive
    en:
    stSysCtlDes = Drive;
    SYM_Current_State=0;
    state SYM_InvrStM
      en,du:
      state Second_State
        state Init
          en,du:
          flgTranDrvInit=1;
        state DrvInit
          en,du:
          flgTranDrvInitToCal=1;
        state Calibration
          state MoCSop
            en,du:
            stSysCtlDes=MoCSop;
          state SensCalFW
            en,du:
            stSysCtlDes=SensCalFW
          state TestPulse
            en,du:
            stSysCtlDes=TestPulse
          (default) -> MoCSop
          SensCalFW -> TestPulse : [flgTranSnsrCalToTestPls]
          MoCSop -> SensCalFW : [flgTranMoCSOPToSnsrCal]
        state FreeWheel
          en,du:
          stSysCtlDes=FreeWheel;
        state alOffsetCalFW
          en,du:
          stSysCtlDes=alOffsetCalFW;
        state Standby
          en,du:
          stSysCtlDes=Standby;
          SYM_flgRunRea=1;
          Standby -> (junction 246) [order 1]
          (junction 246) -> Standby : [stDrvCtlDes==Run]{flgTranStbToCtrl=1}
        state alOffsetCalAcc
          en,du:
          stSysCtlDes=alOffsetCalAcc;
        state Run
          en,du:
          stSysCtlDes=Run;
          flgTranStbToCtrl=1;
          SYM_flgRunRea=0;
          exit:
          SYM_flgRunRea=1;
          Run -> (junction 243) [order 1]
          (junction 243) -> Run : [stDrvCtlDes==Standby]{flgTranStbToCtrl=0}
        (default) -> Init
        (junction 145) -> Init [order 1] : [~flgStbRea]
        Init -> DrvInit : [flgTranDrvInit]
        FreeWheel -> (junction 145) : [~flgTranToFW]
        (junction 145) -> Standby [order 2] : [flgStbRea]
        DrvInit -> Run [order 3] : [flgTranDrvInitToCal ...
            | &&stDrvCtlDes== Run]
        DrvInit -> Standby [order 2] : [flgTranDrvInitToCal ...
            | &&stDrvCtlDes== Standby]
        DrvInit -> Calibration [order 1] : [flgTranDrvInitToCal ...
            | &&stDrvCtlDes== Calibration]
        Second_State -> FreeWheel [order 1] : [flgTranToFW]
        Calibration -> Run [order 1] : [flgTranMoCSOPToRun ...
            | && stDrvCtlDes== Run ]
        Calibration -> Standby [order 2] : [flgTranCalToStb]
        alOffsetCalFW -> Standby [order 1] : [stDrvCtlDes~=alOffsetCalFW]
        Standby -> alOffsetCalFW [order 2] : [stDrvCtlDes==alOffsetCalFW]
        alOffsetCalFW -> alOffsetCalAcc [order 2] : [stDrvCtlDes==alOffsetCalAcc]
        alOffsetCalAcc -> alOffsetCalFW [order 1] : [stDrvCtlDes==alOffsetCalFW]
        Run -> Standby [order 1] : [~flgTranStbToCtrl]
        Standby -> Run [order 1] : [flgTranStbToCtrl]
        Standby -> alOffsetCalAcc [order 3] : [stDrvCtlDes==alOffsetCalAcc]
        alOffsetCalAcc -> Standby [order 2] : [stDrvCtlDes~=alOffsetCalAcc]
      state Failure
        en,du:
        stSysCtlDes=FreeWheel;
      state Discharge
        en,du:
        stSysCtlDes=Discharge;
      (default) -> Second_State
      Failure -> (junction 145) : [flgTranErrToStb]
      Discharge -> (junction 145) : [~flgTranDcha]
      Second_State -> Failure [order 1] : [flgTranToErr]
      SYM_InvrStM -> Discharge [order 1] : [flgTranDcha]
    state SYM_Invrlnp
      en:SYM_Current_State=10;
      state SYM_Invrlnp_Check
        en:SYM_Current_State=11;
      (default) -> SYM_Invrlnp_Check
    (junction 258) -> Drive
    SYM_Invrlnp -> (junction 258) : [ISC_bT15==0]{flgAllwDrv=0}
    SYM_InvrStM -> (junction 258) [order 1] : [ISC_bT15==0]{flgAllwDrv=0}
    (default) -> SYM_Invrlnp
    SYM_Invrlnp_Check -> SYM_InvrStM : [flgCmpIMsg ...
        | && ISC_UdcLnkFlt>10 ...
        | && ISC_UdcLnkFlt<450 ...
        | && ISC_bT15 ...
        | && stSysCtlDes==Drive]
  state SYM_OperInp
    en,du:
    flgAllwDrv=0;
    SYM_Current_State=SYM_OperInp;
  state PreDrive
    en:
    stSysCtlDes = PreDrive;
    flgAllwDrv=1;
    %tiPreActvTi++;
    SYM_Current_State=PreDrive;
  state PostDrive
    en:
    stSysCtlDes=PostDrive;
    SYM_Current_State=PostDrive;
  state ShutDown
    en:
    stSysCtlDes = ShutDown
    SYM_Current_State=ShutDown;
  PostDrive -> PreDrive : [stSysCtrl==PreDrive]
  (default) -> SYM_OperInp
  PreDrive -> Drive [order 1] : [flgInitRdy&& ...
      | flgAllwDrv&& ...
      | flgPreDrvDne&& ...
      | ISC_bT15&& ...
      | after(10,tick)]
  Drive -> PostDrive : [~flgAllwDrv]
  SYM_OperInp -> PreDrive : [ISC_bT15==1 ...
      | | ISC_UdcLnkFlt>60 ...
      | | ISC_n>500 ...
      | | ISC_Is>50]
  PreDrive -> ShutDown [order 2] : [flgAllwDrv&& ...
      | flgPreDrvEx&& ...
      | after(10,tick)]
  ShutDown -> SYM_OperInp : [ISC_bT15==1 ...
      | | ISC_UdcLnkFlt>60 ...
      | | ISC_n>500 ...
      | | ISC_Is>50]
  data: flgStbRea local boolean; flgTranCalToStb local boolean; flgTranDcha local boolean; flgTranDrvInitToCal local boolean; flgTranErrToStb local boolean; flgTranMoCSOPToRun local boolean; flgTranMoCSOPToSnsrCal local boolean; flgTranSnsrCalToTestPls local boolean; flgTranStbToCtrl local boolean; flgTranToErr local boolean; flgTranToFW local boolean; Cif_stSysCtrl input uint8; ISC_UdcLnkFlt input int16; ISC_Is input int16; ISC_n input int16; ISC_bT15 input boolean; flgPostDrvDne input uint8; flgPreDrvDne input uint8; flgPreDrvEx input uint8; stSysCtrl input uint8; flgInitRdy input boolean; flgCmpIMsg input uint8; stDrvCtlDes input uint8; ISC_stAlRtrOfs input uint8; ISC_stDesAlRtrOfsClb input uint8; MCT_stFrwhl input uint8; SYM_stDcha input uint8; SYM_Current_State output uint8; SYM_stDrvCtrl output uint8; SYM_stGateDrv output uint8; SYM_flgRunRea output uint8; SYM_OperInp constant uint8 =1; PreDrive constant uint8 =2; ShutDown constant uint8 =5; Drive constant uint8 =3; SYM_Invrlnp constant uint8 =17; SYM_InvrStM constant uint8 =18; PostDrive constant uint8 =4; stSysCtlDes local uint8; flgAllwDrv local boolean; flgTranDrvInit local boolean; stHvbCntct input uint8; bReadyHv input uint8; Calibration constant uint8 =6; MoCSop constant uint8 =7; SensCalFW constant uint8 =8; TestPulse constant uint8 =9; Standby constant uint8 =10; Run constant uint8 =11; alOffsetCalFW constant uint8 =12; alOffsetCalAcc constant uint8 =13; Failure constant uint8 =14; FreeWheel constant uint8 =15; Discharge constant uint8 =16
